simulink model "UpgradedConveyorBeltMechanism"  (R2023a)
settings: Solver=VariableStepAuto  StartTime=0.0  StopTime=30  RelTol=1e-3
values from neighbouring files (symbols this model uses):
  b = 40.6518    [UpgradedConveyorBeltParameters.m]
  B1 = 0.0042    [UpgradedConveyorBeltParameters.m]
  B2 = 0.0084    [UpgradedConveyorBeltParameters.m]
  J1 = 7e-5    (= 7e-05)    [UpgradedConveyorBeltParameters.m]
  J2 = 8e-5    (= 8e-05)    [UpgradedConveyorBeltParameters.m]
  k1 = 2.6552e5    (= 265520)    [UpgradedConveyorBeltParameters.m]
  k2 = 2.6552e5    (= 265520)    [UpgradedConveyorBeltParameters.m]
  k3 = 11.777e4    (= 117770)    [UpgradedConveyorBeltParameters.m]
  Kb = 23e-3    (= 0.023)    [UpgradedConveyorBeltParameters.m]
  Kt = 23e-3    (= 0.023)    [UpgradedConveyorBeltParameters.m]
  L = 0.1    [UpgradedConveyorBeltParameters.m]
  m = 2    [UpgradedConveyorBeltParameters.m]
  R = 0.71    [UpgradedConveyorBeltParameters.m]
  r = 0.0194    [UpgradedConveyorBeltParameters.m]
undefined symbols (not defined in the file or in its folder): J, Kd, Ke
libraries: fl_lib x20, slpidlib x10, fl_ps_legacy_lib x8, nesl_utility x6, SignalEditorBlockLib x5, ee_lib x2, simulink x1
(part 1 of 2)
settings Model: PacingRate=10  Creator=M3tal  LastModifiedBy=M3tal
settings OptimizationCC: DefaultParameterBehavior=Inlined  EnhancedBackFolding=on  PassReuseOutputArgsThreshold=0  OptimizeBlockOrder=speed  DifferentSizesBufferReuse=on
settings DebuggingCC: ParameterTunabilityLossMsg=error
settings HardwareCC: TargetBitPerPointer=64  TargetBitPerSizeT=64  TargetBitPerPtrDiffT=64  TargetLongLongMode=on  TargetIntDivRoundTo=Zero  TargetEndianess=LittleEndian  TargetWordSize=64  TargetHWDeviceType=MATLAB Host  ProdEqTarget=off
settings SFSimCC: MATLABDynamicMemAlloc=off
settings RTWCC: GenCodeOnly=on
settings CodeAppCC: ForceParamTrailComments=on  OperatorAnnotations=on

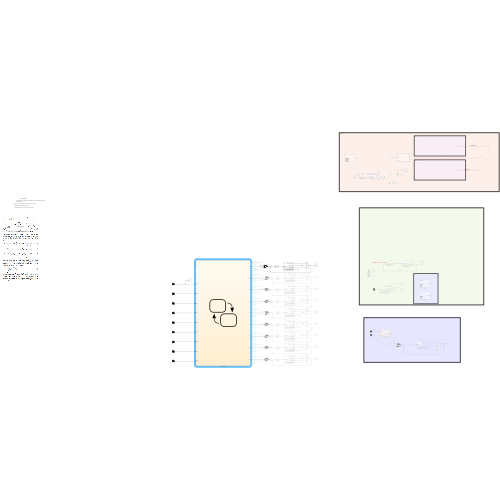
[thumbnail: Simulink's stored preview of the top-level diagram]
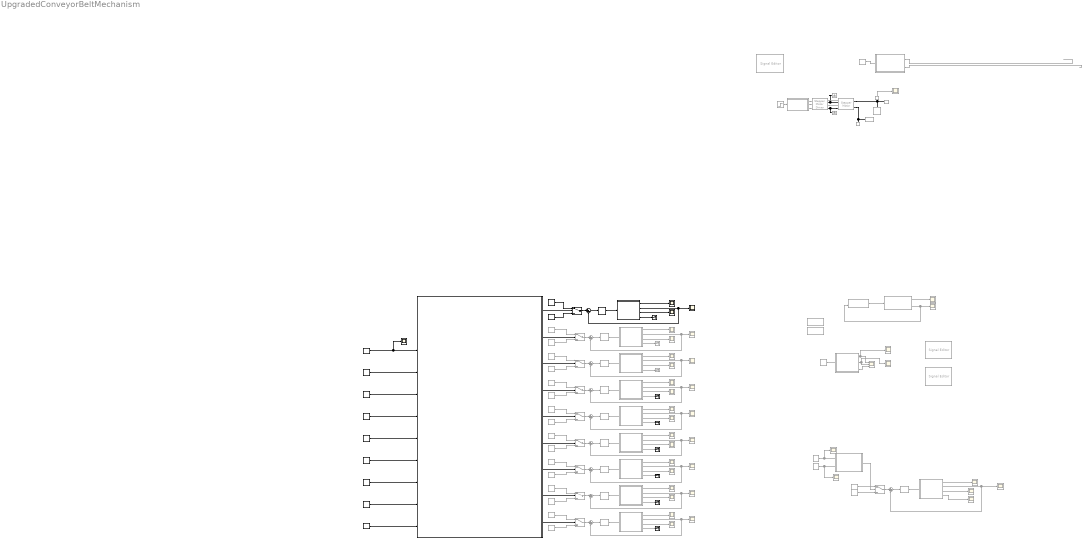
== system UpgradedConveyorBeltMechanism ==
  note: Steppers
  note: X-axis
  note: -replace signals with inports and outports
  note: -record the speed of the dc motor over a period of time
  note: -caluclating the number of steps for each motor for each meal
  note: Y-axis
  note: we using the same mechansim for the steppers that convert the rotational motion to translational motion
  note: m=r*angle in radians
  Belt Mechanism10 : Subsystem  Commented=on
  Constant{,5,7,9,11,13,15,17,19} (9 alike) : Constant  Commented=on  Value=0.2
  Constant{1,6,8,10,12,14,16,18,20} (9 alike) : Constant  Commented=on  Value=0
  Constant2 : Constant  Commented=on
  Constant3 : Constant  Value=0.2
  Constant4 : Constant  Value=0
  Controller : Subsystem  Commented=on  Variant=on  VariantControlMode=label  LabelModeActiveChoice=Position
      settings: AttributesFormatString=%<BlockChoice>
  DC Motor10 : Subsystem  Commented=on
  Demand : Step  Commented=on  Before=10  After=0  SampleTime=0
  ERef A+ : fl_lib/Electrical/Electrical Elements/Electrical Reference  Commented=on
  ERef B- : fl_lib/Electrical/Electrical Elements/Electrical Reference  Commented=on
  Inertia1 : fl_lib/Mechanical/Rotational Elements/Inertia  Commented=on  inertia=0.1 kg*m^2  num_ports=foundation.enum.numPorts2.one  w_specify=off  w_priority=High  w=0 rad/s  w_nominal_specify=off  w_nominal_unit=rad/s  w_nominal_value=1  t_specify=off  t_priority=None  t=0 N*m  t_nominal_specify=off  t_nominal_unit=N*m  t_nominal_value=1
  MATLAB Function : MATLAB Function  Commented=on  TreatAsAtomicUnit=on
  MRRef Motor : fl_lib/Mechanical/Rotational Elements/Mechanical Rotational Reference  Commented=on
  PID Controller{,2..9} (9 alike) : slpidlib/PID Controller  Commented=on  Controller=PID  Form=Parallel  TimeDomain=Continuous-time  UseExternalTs=off  SampleTime=-1  IntegratorMethod=Forward Euler  FilterMethod=Forward Euler  ControllerParametersSource=internal  P=29.8496571480823  I=152.933850283855  UseKiTs=off  D=-0.451147774638306  N=4.48716691500189  UseFilter=on  TunerSelectOption=Transfer Function Based (PID Tuner App)  InitialConditionSource=internal  InitialConditionForIntegrator=0  InitialConditionForFilter=0  DifferentiatorICPrevScaledInput=0  ExternalReset=none  TrackingMode=off  Kt=1  LimitOutput=off  SatLimitsSource=internal  UpperSaturationLimit=inf  LowerSaturationLimit=-inf  LinearizeAsGain=on  AntiWindupMode=none  Kb=1  LimitIntegrator=off  UpperIntegratorSaturationLimit=inf  LowerIntegratorSaturationLimit=-inf  POutMin=[]  POutMax=[]  IOutMin=[]  IOutMax=[]  DOutMin=[]  DOutMax=[]  NOutMin=[]  NOutMax=[]  SumOutMin=[]  SumOutMax=[]  SaturationOutMin=[]  SaturationOutMax=[]  PParamMin=[]  PParamMax=[]  IParamMin=[]  IParamMax=[]  DParamMin=[]  DParamMax=[]  NParamMin=[]  NParamMax=[]  KbParamMin=[]  KbParamMax=[]  KtParamMin=[]  KtParamMax=[]  KbOutMin=[]  KbOutMax=[]  KtOutMin=[]  KtOutMax=[]  IntegratorOutMin=[]  IntegratorOutMax=[]  FilterOutMin=[]  FilterOutMax=[]  SumI1OutMin=[]  SumI1OutMax=[]  SumI2OutMin=[]  SumI2OutMax=[]  SumI3OutMin=[]  SumI3OutMax=[]  SumI4OutMin=[]  SumI4OutMax=[]  SumDOutMin=[]  SumDOutMax=[]  DifferentiatorOutMin=[]  DifferentiatorOutMax=[]  FilterDiffOutCoefMin=[]  FilterDiffOutCoefMax=[]  ReciprocalOutMin=[]  ReciprocalOutMax=[]  SumDenOutMin=[]  SumDenOutMax=[]  SumNumOutMin=[]  SumNumOutMax=[]  DivideOutMin=[]  DivideOutMax=[]  UdiffTsProdOutMin=[]  UdiffTsProdOutMax=[]  NTsProdOutMin=[]  NTsProdOutMax=[]  UintegralTsProdOutMin=[]  UintegralTsProdOutMax=[]  UngainTsProdOutMin=[]  UngainTsProdOutMax=[]  ClampingZeroOutDataTypeStr=Inherit: Inherit via back propagation  ClampingZeroOutMin=[]  ClampingZeroOutMax=[]  FilterDenConstantOutDataTypeStr=Inherit: Inherit via back propagation  FilterDenConstantOutMin=[]  FilterDenConstantOutMax=[]  PCopyOutDataTypeStr=Inherit: Inherit via back propagation  PCopyOutMin=[]  PCopyOutMax=[]  NCopyOutDataTypeStr=Inherit: Inherit via back propagation  NCopyOutMin=[]  NCopyOutMax=[]  IntegratorContinuousStateAttributes=''  IntegratorStateMustResolveToSignalObject=off  IntegratorRTWStateStorageClass=Auto  FilterContinuousStateAttributes=''  FilterStateMustResolveToSignalObject=off  FilterRTWStateStorageClass=Auto  ParallelPVariant=InternalParameters  IdealPVariant=Disabled  IVariant=InternalParameters  DVariant=InternalParameters  IntegratorVariant=Continuous  SatVariant=Disabled  AWVariant=Passthrough  PCopyVariant=Disabled  TRVariant=Disabled  FdbkBlocksVariant=Forward  IdealPFdbkVariant=Disabled  SatFdbkVariant=Disabled  DerivativeFilterVariant=ContFilter  NVariant=InternalParameters  NCopyVariant=Disabled  FilterICVariant=InternalICsFilter  IntegratorICVariant=InternalICs  ExternalResetVariant=Disabled  TRSumVariant=Passthrough  SumFdbkVariant=Disabled  SumVariant=Sum_PID  TsampFilterVariant=InternalTs  TsampNgainVariant=Passthrough  TsampIntegralVariant=Disabled_SignalSpec  ExternalSaturationOutDataTypeStr=Inherit: Same as second input
  PID Controller1 : slpidlib/PID Controller  Controller=PID  Form=Parallel  TimeDomain=Continuous-time  UseExternalTs=off  SampleTime=-1  IntegratorMethod=Forward Euler  FilterMethod=Forward Euler  ControllerParametersSource=internal  P=29.8496571480823  I=152.933850283855  UseKiTs=off  D=-0.451147774638306  N=4.48716691500189  UseFilter=on  TunerSelectOption=Transfer Function Based (PID Tuner App)  InitialConditionSource=internal  InitialConditionForIntegrator=0  InitialConditionForFilter=0  DifferentiatorICPrevScaledInput=0  ExternalReset=none  TrackingMode=off  Kt=1  LimitOutput=off  SatLimitsSource=internal  UpperSaturationLimit=inf  LowerSaturationLimit=-inf  LinearizeAsGain=on  AntiWindupMode=none  Kb=1  LimitIntegrator=off  UpperIntegratorSaturationLimit=inf  LowerIntegratorSaturationLimit=-inf  POutMin=[]  POutMax=[]  IOutMin=[]  IOutMax=[]  DOutMin=[]  DOutMax=[]  NOutMin=[]  NOutMax=[]  SumOutMin=[]  SumOutMax=[]  SaturationOutMin=[]  SaturationOutMax=[]  PParamMin=[]  PParamMax=[]  IParamMin=[]  IParamMax=[]  DParamMin=[]  DParamMax=[]  NParamMin=[]  NParamMax=[]  KbParamMin=[]  KbParamMax=[]  KtParamMin=[]  KtParamMax=[]  KbOutMin=[]  KbOutMax=[]  KtOutMin=[]  KtOutMax=[]  IntegratorOutMin=[]  IntegratorOutMax=[]  FilterOutMin=[]  FilterOutMax=[]  SumI1OutMin=[]  SumI1OutMax=[]  SumI2OutMin=[]  SumI2OutMax=[]  SumI3OutMin=[]  SumI3OutMax=[]  SumI4OutMin=[]  SumI4OutMax=[]  SumDOutMin=[]  SumDOutMax=[]  DifferentiatorOutMin=[]  DifferentiatorOutMax=[]  FilterDiffOutCoefMin=[]  FilterDiffOutCoefMax=[]  ReciprocalOutMin=[]  ReciprocalOutMax=[]  SumDenOutMin=[]  SumDenOutMax=[]  SumNumOutMin=[]  SumNumOutMax=[]  DivideOutMin=[]  DivideOutMax=[]  UdiffTsProdOutMin=[]  UdiffTsProdOutMax=[]  NTsProdOutMin=[]  NTsProdOutMax=[]  UintegralTsProdOutMin=[]  UintegralTsProdOutMax=[]  UngainTsProdOutMin=[]  UngainTsProdOutMax=[]  ClampingZeroOutDataTypeStr=Inherit: Inherit via back propagation  ClampingZeroOutMin=[]  ClampingZeroOutMax=[]  FilterDenConstantOutDataTypeStr=Inherit: Inherit via back propagation  FilterDenConstantOutMin=[]  FilterDenConstantOutMax=[]  PCopyOutDataTypeStr=Inherit: Inherit via back propagation  PCopyOutMin=[]  PCopyOutMax=[]  NCopyOutDataTypeStr=Inherit: Inherit via back propagation  NCopyOutMin=[]  NCopyOutMax=[]  IntegratorContinuousStateAttributes=''  IntegratorStateMustResolveToSignalObject=off  IntegratorRTWStateStorageClass=Auto  FilterContinuousStateAttributes=''  FilterStateMustResolveToSignalObject=off  FilterRTWStateStorageClass=Auto  ParallelPVariant=InternalParameters  IdealPVariant=Disabled  IVariant=InternalParameters  DVariant=InternalParameters  IntegratorVariant=Continuous  SatVariant=Disabled  AWVariant=Passthrough  PCopyVariant=Disabled  TRVariant=Disabled  FdbkBlocksVariant=Forward  IdealPFdbkVariant=Disabled  SatFdbkVariant=Disabled  DerivativeFilterVariant=ContFilter  NVariant=InternalParameters  NCopyVariant=Disabled  FilterICVariant=InternalICsFilter  IntegratorICVariant=InternalICs  ExternalResetVariant=Disabled  TRSumVariant=Passthrough  SumFdbkVariant=Disabled  SumVariant=Sum_PID  TsampFilterVariant=InternalTs  TsampNgainVariant=Passthrough  TsampIntegralVariant=Disabled_SignalSpec  ExternalSaturationOutDataTypeStr=Inherit: Same as second input
  Pulse Generator : DiscretePulseGenerator  Commented=on  PulseType=Time based  Period=40  PhaseDelay=20
  Pulse Generator1 : DiscretePulseGenerator  Commented=on  PulseType=Time based  Period=50  PhaseDelay=5
  Pulse Generator{3..10} (8 alike) : DiscretePulseGenerator  PulseType=Time based  Amplitude=0  Period=50  PhaseDelay=5
  Pulse Generator11 : DiscretePulseGenerator  Commented=on  PulseType=Time based  Amplitude=12  Period=11  PulseWidth=50  PhaseDelay=2
  Pulse Generator2 : DiscretePulseGenerator  PulseType=Time based  Period=50  PulseWidth=50  PhaseDelay=25
  Scope{,1..3,8..22,24..38} (34 alike) : Scope  Commented=on
  Scope23 : Scope  Commented=on  NumInputPorts=3
  Scope{4..7} (4 alike) : Scope
  Sensing Angle : Subsystem  Commented=on
      mask Display: disp('a')
  Sensor : SignalEditorBlockLib/Signal Editor  Commented=on  FileName=Crane_Sensor.mat  ActiveScenario=Scenario  ActiveSignal=Crane signal  IsBus=off  OutputBusObjectStr=Bus: BusObject  SampleTime=0  Interpolate=off  ZeroCross=off  OutputAfterFinalValue=Setting to zero  Unit=inherit  PreserveSignalName=on  ApplySigPropsToAllScenarios=on
  Sensor1 : SignalEditorBlockLib/Signal Editor  Commented=on  FileName=Belt_Sensor.mat  ActiveScenario=Scenario  ActiveSignal=Belt Signal  IsBus=off  OutputBusObjectStr=Bus: BusObject  SampleTime=0  Interpolate=off  ZeroCross=off  OutputAfterFinalValue=Setting to zero  Unit=inherit  PreserveSignalName=on  ApplySigPropsToAllScenarios=on
  Sensors : Stateflow chart  Commented=on  TreatAsAtomicUnit=on
  Sensors Logic : Stateflow chart  TreatAsAtomicUnit=on
      settings: PortSchema="{\"entries\":[{\"content\":{\"sides\":[{\"content\":{\"connectorIds\":[\"In10\",\"In11\",\"In1\",\"In2\",\"In3\",\"In4\",\"In5\",\"In6\",\"In7\",\"In8\",\"In9\"]},\"type\":\"ConnectorPlacement.EquallySpacedRectSide\",\"uuid\":\"dd9ce701-3689-4654-9b21-5529dab0541a\"},{\"content\":{\"connectorIds\":[\"Out1\",\"Out2\",\"Out3\",\"Out4\",\"Out5\",\"Out6\",\"Out7\",\"Out8\",\"Out9\"],\"side\":\"RIGHT\"},\"type\":\"ConnectorPlacement.EquallySpacedRectSide\",\"uuid\":\"ff8f0f67-846c-4703-aeda-d87216d47c92\"},{\"content\":{\"side\":\"TOP\"},\"type\":\"ConnectorPlacement.EquallySpacedRectSide\",\"uuid\":\"ae968bb7-da0f-44fd-802b-06f57922bbce\"}]},\"type\":\"ConnectorPlacement.EquallySpacedConnector\",\"uuid\":\"820653e5-881f-4b8b-9810-894dc5dde637\"}],\"packageUris\":[\"http://schema.mathworks.com/mf0/Connector/R2020b\"],\"version\":\"1.0\"}"
  Shaft Angle : Scope  Commented=on
  Shaft Free End : fl_lib/Mechanical/Rotational Elements/Rotational Free End  Commented=on  w_specify=off  w_priority=None  w=0 rad/s  w_nominal_specify=off  w_nominal_unit=rad/s  w_nominal_value=1
  Signal Editor : SignalEditorBlockLib/Signal Editor  Commented=on  FileName=X_Position.mat  ActiveScenario=Scenario  ActiveSignal=X  IsBus=off  OutputBusObjectStr=Bus: BusObject  SampleTime=0  Interpolate=off  ZeroCross=off  OutputAfterFinalValue=Setting to zero  Unit=inherit  PreserveSignalName=on  ApplySigPropsToAllScenarios=on
  Signal Editor1 : SignalEditorBlockLib/Signal Editor  Commented=on  FileName=Y_Position.mat  ActiveScenario=Scenario  ActiveSignal=Y  IsBus=off  OutputBusObjectStr=Bus: BusObject  SampleTime=0  Interpolate=off  ZeroCross=off  OutputAfterFinalValue=Setting to zero  Unit=inherit  PreserveSignalName=on  ApplySigPropsToAllScenarios=on
  Signal Editor2 : SignalEditorBlockLib/Signal Editor  Commented=on  FileName=untitled.mat  ActiveScenario=Scenario  ActiveSignal=Signal 1  IsBus=off  OutputBusObjectStr=Bus: BusObject  SampleTime=0  Interpolate=off  ZeroCross=off  OutputAfterFinalValue=Setting to zero  Unit=inherit  PreserveSignalName=on  ApplySigPropsToAllScenarios=on
  Solver Configuration : nesl_utility/Solver Configuration  Commented=on  PhysicalDomain=network_engine_domain  SubClassName=solver  LeftPortType=input  RightPortType=generic  Tones=[]  Harmonics=[]  SimulateNoise=off  Profile=off  UseLocalSampling=off  EnableSwitchedLinearOptims=on  FrequencyDomain=off  UseCCode=off  RelTol=0.001  AbsTol=1e-06  MinStep=1e-09  ToWorkspace=off  RevertToSquareIcSolve=off  NumHomotopyIterations=100  PhasorMode=off  PhasorModeNumHarmonics=1  ConsistencySolver=NEWTON_FTOL  IndexReductionMethod=DerivativeReplacement  DoDC=off  ResidualTolerance=1e-9  ConsistencyTolSource=GLOBAL  ConsistencyAbsTol=0.001  ConsistencyRelTol=0.001  ConsistencyTolFactor=0.001  UseLocalSolver=off  LocalSolverChoice=NE_BACKWARD_EULER_ADVANCER  ResolveIndetEquations=on  FunctionEvalNumThread=1  LocalSolverSampleTime=.001  DoFixedCost=off  MaxNonlinIter=3  MaxModeIter=2  ComputeImpulses=off  ImpulseIterations=2  LinearAlgebra=auto  LinearAlgebraNumThread=0  EquationFormulation=NE_TIME_EF  DelaysMemoryBudget=1024  AutomaticFiltering=on  FilteringTimeConstant=0.001  PartitionStorageMethod=AS_NEEDED  PartitionMemoryBudget=1024  PartitionMethod=FAST
  Stepper Motor : ee_lib/Electromechanical/Reluctance & Stepper/Stepper Motor  Commented=on  step_or_av=ee.enum.electromech.simulationMode.stepping  Ra=1.3 Ohm  La=2.9 mH  Km=0.315 N*m/A  Td=25 mN*m  Rm=Inf Ohm  w_vec=[ 0 1000 3e+3 ] rpm  T_vec=[ 2 2 1 ] N*m  assert_if_slipping=0  J_total=1e-4 kg*m^2  max_step_rate=10 Hz  Step=1.8 deg  J=82 g*cm^2  B=1e-2 N*m/(rad/s)  speed0=0 rpm  theta0=0 deg  alpha=[.00393, .00393] 1/K  Tmeas=25 degC  Tmeas2=125 degC  T_vec2=[1.7, 1.7, .85] N*m  half_stepping=ee.enum.electromech.steppingModeAveraged.fullStep  thermal_masses=[100, 100] J/K  initial_temperatures=[25, 25] degC  rotor_thermal_mass=50 J/K  rotor_initial_temperature=25 degC  Rm_percent_rotor=90
      settings: InternalSimscapePortConfiguration="{\"Bottom\":[],\"Left\":[{\"id\":\"pA\",\"label\":\"A+\",\"type\":\"foundation.electrical.electrical\"},{\"id\":\"nA\",\"label\":\"A-\",\"type\":\"foundation.electrical.electrical\"},{\"id\":\"pB\",\"label\":\"B+\",\"type\":\"foundation.electrical.electrical\"},{\"id\":\"nB\",\"label\":\"B-\",\"type\":\"foundation.electrical.electrical\"}],\"Right\":[{\"id\":\"R\",\"label\":\"R\",\"type\":\"foundation.mechanical.rotational.rotational\"},{\"id\":\"C\",\"label\":\"C\",\"type\":\"foundation.mechanical.rotational.rotational\"}],\"Top\":[]}"
  Stepper Motor Driver : ee_lib/Electromechanical/Reluctance & Stepper/Stepper Motor Driver  Commented=on  step_or_av=1  step_rate_per_volt=10 Hz/V  Venable=2.5 V  Vreverse=2.5 V  supply_ports=ee.enum.supply_ports.hidesupply  Vm=5 V  Vsupply=10 V  half_stepping=0  stepping_mode=ee.enum.electromech.steppingMode.fullStep  numMicroSteps=4  Im=1.2 A
      settings: InternalSimscapePortConfiguration="{\"Bottom\":[],\"Left\":[{\"id\":\"ENA\",\"label\":\"ENA\",\"type\":\"foundation.electrical.electrical\"},{\"id\":\"REF\",\"label\":\"REF\",\"type\":\"foundation.electrical.electrical\"},{\"id\":\"REV\",\"label\":\"REV\",\"type\":\"foundation.electrical.electrical\"}],\"Right\":[{\"id\":\"pA\",\"label\":\"A+\",\"type\":\"foundation.electrical.electrical\"},{\"id\":\"nA\",\"label\":\"A-\",\"type\":\"foundation.electrical.electrical\"},{\"id\":\"pB\",\"label\":\"B+\",\"type\":\"foundation.electrical.electrical\"},{\"id\":\"nB\",\"label\":\"B-\",\"type\":\"foundation.electrical.electrical\"}],\"Top\":[]}"
  Subsystem : Subsystem  Commented=on
  Subsystem1 : Subsystem  Commented=on
  Subsystem10 : Subsystem  Commented=on
  Subsystem2 : Subsystem
  Subsystem3 : Subsystem  Commented=on
  Subsystem4 : Subsystem  Commented=on
  Subsystem5 : Subsystem  Commented=on
  Subsystem6 : Subsystem  Commented=on
  Subsystem7 : Subsystem  Commented=on
  Subsystem8 : Subsystem  Commented=on
  Subsystem9 : Subsystem  Commented=on
  Sum{,2..9} (9 alike) : Sum  Commented=on  Inputs=|+-
  Sum1 : Sum  Inputs=|+-
  Switch{,2..9} (9 alike) : Switch  Commented=on  Criteria=u2 ~= 0  Threshold=1  SaturateOnIntegerOverflow=off  InputSameDT=off
  Switch1 : Switch  Criteria=u2 ~= 0  Threshold=1  SaturateOnIntegerOverflow=off  InputSameDT=off
  Terminator{,3..8} (7 alike) : Terminator
  Terminator1 : Terminator  Commented=on
  Terminator2 : Terminator  Commented=on
  wires:
  Pulse Generator1/1 -> Scope/1, Sensors/1(Crane)
  Subsystem1/2(load velocity) -> Sum/2, Scope2/1  "Velocity"
  Pulse Generator/1 -> Scope3/1, Sensors/2(Belt)
  Subsystem/1(drive pulley velocity) -> Scope25/1, Scope23/1
  Subsystem/2(load velocity) -> Scope23/2, Scope24/1
  Subsystem/3(driven pulley velocity) -> Scope23/3
  Pulse Generator11/1 -> Subsystem/1(Voltage)
  Sum/1 -> PID Controller/1
  Sensors/1(Voltage) -> Switch/2
  Constant1/1 -> Switch/3
  PID Controller/1 -> Subsystem1/1(Voltage)
  Switch/1 -> Sum/1
  Constant/1 -> Switch/1
  Subsystem1/1(drive pulley velocity) -> Scope26/1
  Subsystem1/4(driven pulley Velocity) -> Scope27/1
  Subsystem1/3(load position) -> Scope1/1
  Pulse Generator5/1 -> Sensors Logic/4(Belt4)
  Pulse Generator9/1 -> Sensors Logic/8(Belt8)
  Pulse Generator7/1 -> Sensors Logic/6(Belt6)
  Pulse Generator2/1 -> Scope4/1, Sensors Logic/1(Belt1)
  Pulse Generator8/1 -> Sensors Logic/7(Belt7)
  Pulse Generator3/1 -> Sensors Logic/2(Belt2)
  Pulse Generator6/1 -> Sensors Logic/5(Belt5)
  Pulse Generator10/1 -> Sensors Logic/9(Belt9)
  Pulse Generator4/1 -> Sensors Logic/3(Belt3)
  Constant2/1 -> MATLAB Function/1(meal)
  ? -> DC Motor10/1(Voltage)
  Belt Mechanism10/2(Velocity) -> Scope29/1, DC Motor10/2(Velocity)  "Velocity"
  Belt Mechanism10/1(Position) -> Scope28/1
  DC Motor10/1(Tourque) -> Belt Mechanism10/1(Tourque)  "Tourque"
  Subsystem2/1(drive pulley velocity) -> Scope7/1
  Sum1/1 -> PID Controller1/1
  Switch1/1 -> Sum1/1
  Constant3/1 -> Switch1/1
  Constant4/1 -> Switch1/3
  PID Controller1/1 -> Subsystem2/1(Voltage)
  Subsystem2/2(load velocity) -> Sum1/2, Scope6/1  "Velocity"
  Subsystem2/3(load position) -> Scope5/1
  Subsystem2/4(driven pulley Velocity) -> Terminator/1
  Sensors Logic/1(V1) -> Switch1/2
  Subsystem3/3(load position) -> Scope8/1
  Sensors Logic/2(V2) -> Switch2/2
  Sum2/1 -> PID Controller2/1
  Constant6/1 -> Switch2/3
  Subsystem3/1(drive pulley velocity) -> Scope10/1
  Subsystem3/2(load velocity) -> Sum2/2, Scope9/1  "Velocity"
  PID Controller2/1 -> Subsystem3/1(Voltage)
  Constant5/1 -> Switch2/1
  Switch2/1 -> Sum2/1
  Subsystem3/4(driven pulley Velocity) -> Terminator1/1
  Subsystem4/4(driven pulley Velocity) -> Terminator2/1
  Sum3/1 -> PID Controller3/1
  Constant8/1 -> Switch3/3
  Subsystem4/2(load velocity) -> Sum3/2, Scope13/1  "Velocity"
  Switch3/1 -> Sum3/1
  Constant7/1 -> Switch3/1
  PID Controller3/1 -> Subsystem4/1(Voltage)
  Subsystem4/3(load position) -> Scope12/1
  Subsystem4/1(drive pulley velocity) -> Scope11/1
  Sensors Logic/3(V3) -> Switch3/2
  Subsystem5/4(driven pulley Velocity) -> Terminator3/1
  Sum4/1 -> PID Controller4/1
  Constant10/1 -> Switch4/3
  Subsystem5/2(load velocity) -> Sum4/2, Scope16/1  "Velocity"
  Switch4/1 -> Sum4/1
  Constant9/1 -> Switch4/1
  PID Controller4/1 -> Subsystem5/1(Voltage)
  Subsystem5/3(load position) -> Scope15/1
  Subsystem5/1(drive pulley velocity) -> Scope14/1
  Sensors Logic/4(V4) -> Switch4/2
  Subsystem6/4(driven pulley Velocity) -> Terminator4/1
  Sum5/1 -> PID Controller5/1
  Constant12/1 -> Switch5/3
  Subsystem6/2(load velocity) -> Sum5/2, Scope19/1  "Velocity"
  Switch5/1 -> Sum5/1
  Constant11/1 -> Switch5/1
  PID Controller5/1 -> Subsystem6/1(Voltage)
  Subsystem6/3(load position) -> Scope18/1
  Subsystem6/1(drive pulley velocity) -> Scope17/1
  Sensors Logic/5(V5) -> Switch5/2
  Sensors Logic/6(V6) -> Switch6/2
  Subsystem7/1(drive pulley velocity) -> Scope20/1
  Subsystem7/2(load velocity) -> Sum6/2, Scope22/1  "Velocity"
  Subsystem7/3(load position) -> Scope21/1
  Subsystem7/4(driven pulley Velocity) -> Terminator5/1
  Constant13/1 -> Switch6/1
  Switch6/1 -> Sum6/1
  Constant14/1 -> Switch6/3
  Sum6/1 -> PID Controller6/1
  PID Controller6/1 -> Subsystem7/1(Voltage)
  Sensors Logic/7(V7) -> Switch7/2
  Subsystem8/1(drive pulley velocity) -> Scope30/1
  Sum7/1 -> PID Controller7/1
  Constant16/1 -> Switch7/3
  Subsystem8/2(load velocity) -> Sum7/2, Scope32/1  "Velocity"
  Subsystem8/4(driven pulley Velocity) -> Terminator6/1
  Constant15/1 -> Switch7/1
  Subsystem8/3(load position) -> Scope31/1
  Switch7/1 -> Sum7/1
  PID Controller7/1 -> Subsystem8/1(Voltage)
  PID Controller8/1 -> Subsystem9/1(Voltage)
  Switch8/1 -> Sum8/1
  Constant17/1 -> Switch8/1
  Subsystem9/3(load position) -> Scope34/1
  Subsystem9/1(drive pulley velocity) -> Scope33/1
  Subsystem9/4(driven pulley Velocity) -> Terminator7/1
  Sum8/1 -> PID Controller8/1
  Subsystem9/2(load velocity) -> Sum8/2, Scope35/1  "Velocity"
  Sensors Logic/8(V8) -> Switch8/2
  Constant18/1 -> Switch8/3
  Subsystem10/2(load velocity) -> Sum9/2, Scope38/1  "Velocity"
  Constant20/1 -> Switch9/3
  Subsystem10/1(drive pulley velocity) -> Scope36/1
  Subsystem10/3(load position) -> Scope37/1
  Subsystem10/4(driven pulley Velocity) -> Terminator8/1
  Sum9/1 -> PID Controller9/1
  PID Controller9/1 -> Subsystem10/1(Voltage)
  Sensors Logic/9(V9) -> Switch9/2
  Switch9/1 -> Sum9/1
  Constant19/1 -> Switch9/1
  ? -> ?  "XTheta (degrees)"
  ? -> ?  "YTheta (degrees)"
  Demand/1 -> Controller/1(Ref)
  Sensing Angle/1(theta) -> Shaft Angle/1
  MATLAB Function/1(x) -> ?
  MATLAB Function/2(y) -> ?
  connections:
  MRRef Motor/LConn1 -- Stepper Motor/RConn2 -- Solver Configuration/RConn1
  Stepper Motor/LConn4 -- Stepper Motor Driver/RConn4 -- ERef B-/LConn1
  Stepper Motor Driver/RConn2 -- Stepper Motor/LConn2 -- ERef A+/LConn1
  Sensing Angle/LConn1 -- Stepper Motor/RConn1 -- Inertia1/LConn1 -- Shaft Free End/LConn1
  Stepper Motor Driver/RConn1 -- Stepper Motor/LConn1
  Controller/RConn2 -- Stepper Motor Driver/LConn2
  Controller/RConn3 -- Stepper Motor Driver/LConn3
  Controller/RConn1 -- Stepper Motor Driver/LConn1
  Stepper Motor Driver/RConn3 -- Stepper Motor/LConn3

== system UpgradedConveyorBeltMechanism/Belt Mechanism10 ==
  note: Note: The term $K \frac{d\theta}{dt}$ ​ represents a damping torque that is proportional to the angular velocity
  note: $\frac{d^2\theta}{dt^2} = \frac{1}{J} \left(T - K \frac{d\theta}{dt}\right)$
      | belt mechanism equaition based on newton seconed law for rotational motion
  Tourque : Inport
  Gain1 : Gain  Gain=1/J
  Integrator2 : Integrator
  Integrator3 : Integrator
  Subtract : Sum  Inputs=+-
  damping coefficient : Gain  Gain=Kd
  Position : Outport
  Velocity : Outport  Port=2
  wires:
  Integrator2/1 -> damping coefficient/1, Velocity/1, Integrator3/1  "Velocity"
  Tourque/1 -> Subtract/1
  Subtract/1 -> Gain1/1
  Integrator3/1 -> Position/1  "Position"
  damping coefficient/1 -> Subtract/2
  Gain1/1 -> Integrator2/1  "theta_dot_dot"

== system UpgradedConveyorBeltMechanism/Controller ==
  Ref : Inport
  Position : Subsystem  VariantControl=Position
  Speed : Subsystem  VariantControl=Speed
  PWM : PMIOPort  Side=Right
  0v : PMIOPort  Port=2  Side=Right
  REV : PMIOPort  Port=3  Side=Right

== system UpgradedConveyorBeltMechanism/DC Motor10 ==
  note: Armature Controlled DC Motor
      |
      | $E_a = R_a \cdot I_a + L_a \cdot \frac{di_a}{dt} + K_b \cdot \frac{d\theta}{dt}$
      | $T_{m} = K_{t} \cdot I_{a}$
  Voltage : Inport
  Velocity : Inport  Port=2
  Constant1 : Constant  Value=R
  Gain1 : Gain  Gain=Kb
  Gain2 : Gain  Gain=1/L
  Gain3 : Gain  Gain=Kt
  Integrator : Integrator
  Product : Product
  Subtract : Sum  Inputs=+--
  Tourque : Outport
  wires:
  Voltage/1 -> Subtract/1
  Integrator/1 -> Product/1, Gain3/1  "i"
  Gain3/1 -> Tourque/1
  Gain1/1 -> Subtract/2
  Velocity/1 -> Gain1/1
  Constant1/1 -> Product/2
  Product/1 -> Subtract/3
  Gain2/1 -> Integrator/1  "i_dot"
  Subtract/1 -> Gain2/1

== system UpgradedConveyorBeltMechanism/Sensing Angle ==
  MRRef : fl_lib/Mechanical/Rotational Elements/Mechanical Rotational Reference
  Motion Sensor : fl_lib/Mechanical/Mechanical Sensors/Ideal Rotational Motion Sensor  reference=foundation.enum.MeasurementReference.difference  acceleration_port=false  velocity_port=true  position_port=true  wrap_angle=simscape.enum.onoff.off  offset=0 rad
  deg : nesl_utility/PS-Simulink Converter  PhysicalDomain=network_engine_domain  SubClassName=ps_output  LeftPortType=input  RightPortType=output  PseudoPeriodic=off  Frequencies=[]  VectorFormat=1-D array  Unit=deg  AffineConversion=off
  R : PMIOPort  Side=Left
  theta : Outport  VectorParamsAs1DForOutWhenUnconnected=off
  wires:
  deg/1 -> theta/1
  connections:
  R/RConn1 -- Motion Sensor/LConn1
  Motion Sensor/RConn3 -- deg/LConn1
  MRRef/LConn1 -- Motion Sensor/RConn1

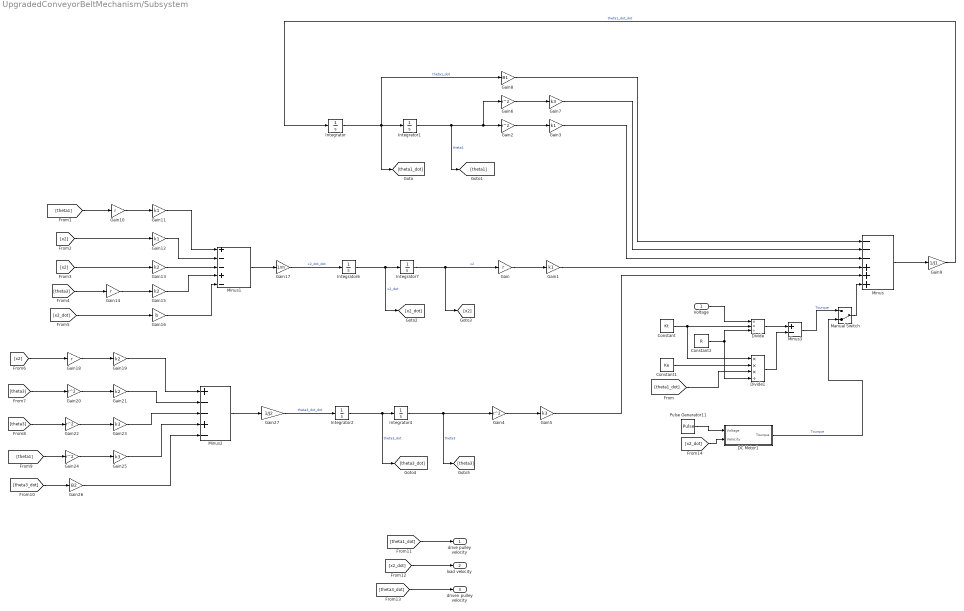
== system UpgradedConveyorBeltMechanism/Subsystem ==
  Voltage : Inport
  Constant : Constant  Value=Kt
  Constant1 : Constant  Value=Ke
  Constant2 : Constant  Value=R
  DC Motor1 : Subsystem
  Divide : Product  Inputs=**/
  Divide1 : Product  Inputs=***/
  Gain{,10,14,18} (4 alike) : Gain  Gain=r
  Gain{1,3,11..12} (4 alike) : Gain  Gain=k1
  Gain{13,15,19,21} (4 alike) : Gain  Gain=k2
  Gain16 : Gain  Gain=b
  Gain17 : Gain  Gain=1/m
  Gain{2,4,6,20,22,24} (6 alike) : Gain  Gain=r^2
  Gain{5,7,23,25} (4 alike) : Gain  Gain=k3
  Gain26 : Gain  Gain=B2
  Gain27 : Gain  Gain=1/J2
  Gain8 : Gain  Gain=B1
  Gain9 : Gain  Gain=1/J1
  Integrator{,1..2,4,6..7} (6 alike) : Integrator
  Manual Switch : ManualSwitch  CurrentSetting=0
  Minus : Sum  Inputs=---+++
  Minus1 : Sum  Inputs=+--+-
  Minus2 : Sum  Inputs=+--+-
  Minus3 : Sum  Inputs=+-
  Pulse Generator11 : DiscretePulseGenerator  PulseType=Time based  Amplitude=12  Period=11  PulseWidth=50  PhaseDelay=2
  drive pulley velocity : Outport
  load velocity : Outport  Port=2
  driven pulley velocity : Outport  Port=3
  wires:
  Gain23/1 -> Minus2/3
  Gain4/1 -> Gain5/1
  [theta1] -> Gain24/1
  Gain11/1 -> Minus1/1
  [theta3_dot] -> Gain26/1
  Gain26/1 -> Minus2/5
  Gain22/1 -> Gain23/1
  Gain19/1 -> Minus2/1
  Gain21/1 -> Minus2/2
  Integrator/1 -> Integrator1/1, [theta1_dot], Gain8/1  "theta1_dot"
  Integrator1/1 -> Gain6/1, Gain2/1, [theta1]  "theta1"
  Integrator6/1 -> Integrator7/1, [x2_dot]  "x2_dot"
  Gain3/1 -> Minus/3
  Gain18/1 -> Gain19/1
  Gain1/1 -> Minus/4
  Gain2/1 -> Gain3/1
  Integrator2/1 -> [theta3_dot], Integrator4/1  "theta3_dot"
  Integrator4/1 -> Gain4/1, [theta3]  "theta3"
  [x2] -> Gain12/1
  Gain/1 -> Gain1/1
  Gain10/1 -> Gain11/1
  [theta1_dot] -> Divide1/3
  Gain24/1 -> Gain25/1
  Gain13/1 -> Minus1/3
  [theta3] -> Gain20/1
  [theta3] -> Gain14/1
  Gain15/1 -> Minus1/4
  Gain6/1 -> Gain7/1
  [theta3] -> Gain22/1
  Gain5/1 -> Minus/5
  [theta1] -> Gain10/1
  [x2] -> Gain18/1
  Minus2/1 -> Gain27/1
  Minus1/1 -> Gain17/1
  Minus/1 -> Gain9/1
  Gain7/1 -> Minus/2
  Integrator7/1 -> Gain/1, [x2]  "x2"
  Gain16/1 -> Minus1/5
  Gain8/1 -> Minus/1
  Gain17/1 -> Integrator6/1  "x2_dot_dot"
  Gain14/1 -> Gain15/1
  Gain20/1 -> Gain21/1
  Gain9/1 -> Integrator/1  "theta1_dot_dot"
  Gain12/1 -> Minus1/2
  Gain25/1 -> Minus2/4
  [x2] -> Gain13/1
  Minus3/1 -> Manual Switch/1  "Tourque"
  [x2_dot] -> Gain16/1
  [theta1_dot] -> drive pulley velocity/1
  [x2_dot] -> load velocity/1
  [theta3_dot] -> driven pulley velocity/1
  Gain27/1 -> Integrator2/1  "theta3_dot_dot"
  Voltage/1 -> Divide/1
  Constant/1 -> Divide/2, Divide1/1
  Constant2/1 -> Divide1/4, Divide/3
  Divide/1 -> Minus3/1
  Constant1/1 -> Divide1/2
  Divide1/1 -> Minus3/2
  Manual Switch/1 -> Minus/6
  DC Motor1/1(Tourque) -> Manual Switch/2  "Tourque"
  Pulse Generator11/1 -> DC Motor1/1(Voltage)
  [x2_dot] -> DC Motor1/2(Velocity)

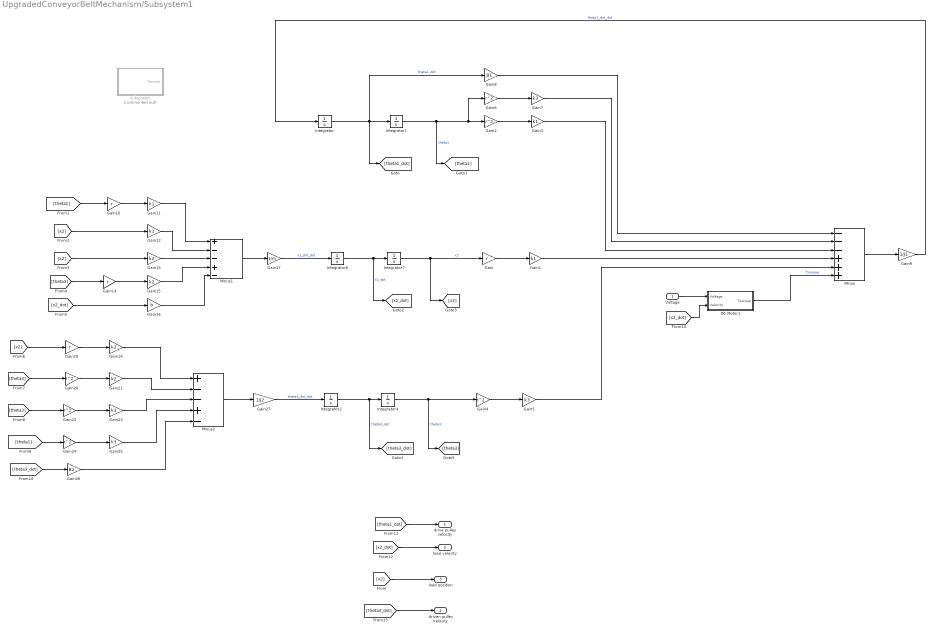
== system UpgradedConveyorBeltMechanism/Subsystem1 ==
  Voltage : Inport
  DC Motor1 : Subsystem
  Gain{,10,14,18} (4 alike) : Gain  Gain=r
  Gain{1,3,11..12} (4 alike) : Gain  Gain=k1
  Gain{13,15,19,21} (4 alike) : Gain  Gain=k2
  Gain16 : Gain  Gain=b
  Gain17 : Gain  Gain=1/m
  Gain{2,4,6,20,22,24} (6 alike) : Gain  Gain=r^2
  Gain{5,7,23,25} (4 alike) : Gain  Gain=k3
  Gain26 : Gain  Gain=B2
  Gain27 : Gain  Gain=1/J2
  Gain8 : Gain  Gain=B1
  Gain9 : Gain  Gain=1/J1
  Integrator{,1..2,4,6..7} (6 alike) : Integrator
  Minus : Sum  Inputs=---+++
  Minus1 : Sum  Inputs=+--+-
  Minus2 : Sum  Inputs=+--+-
  Subsystem : Subsystem  Commented=on
  drive pulley velocity : Outport
  load velocity : Outport  Port=2
  load position : Outport  Port=3
  driven pulley Velocity : Outport  Port=4
  wires:
  Gain23/1 -> Minus2/3
  Gain4/1 -> Gain5/1
  [theta1] -> Gain24/1
  Gain11/1 -> Minus1/1
  [theta3_dot] -> Gain26/1
  Gain26/1 -> Minus2/5
  Gain22/1 -> Gain23/1
  Gain19/1 -> Minus2/1
  Gain21/1 -> Minus2/2
  Integrator/1 -> Integrator1/1, [theta1_dot], Gain8/1  "theta1_dot"
  Integrator1/1 -> Gain6/1, Gain2/1, [theta1]  "theta1"
  Integrator6/1 -> Integrator7/1, [x2_dot]  "x2_dot"
  Gain3/1 -> Minus/3
  Gain18/1 -> Gain19/1
  Gain1/1 -> Minus/4
  Gain2/1 -> Gain3/1
  Integrator2/1 -> [theta3_dot], Integrator4/1  "theta3_dot"
  Integrator4/1 -> Gain4/1, [theta3]  "theta3"
  [x2] -> Gain12/1
  Gain/1 -> Gain1/1
  Gain10/1 -> Gain11/1
  Gain24/1 -> Gain25/1
  Gain13/1 -> Minus1/3
  [theta3] -> Gain20/1
  [theta3] -> Gain14/1
  Gain15/1 -> Minus1/4
  Gain6/1 -> Gain7/1
  [theta3] -> Gain22/1
  Gain5/1 -> Minus/5
  [theta1] -> Gain10/1
  [x2] -> Gain18/1
  Minus2/1 -> Gain27/1
  Minus1/1 -> Gain17/1
  Minus/1 -> Gain9/1
  Gain7/1 -> Minus/2
  Integrator7/1 -> Gain/1, [x2]  "x2"
  Gain16/1 -> Minus1/5
  Gain8/1 -> Minus/1
  Gain17/1 -> Integrator6/1  "x2_dot_dot"
  Gain14/1 -> Gain15/1
  Gain20/1 -> Gain21/1
  Gain9/1 -> Integrator/1  "theta1_dot_dot"
  Gain12/1 -> Minus1/2
  Gain25/1 -> Minus2/4
  [x2] -> Gain13/1
  [x2_dot] -> Gain16/1
  [theta1_dot] -> drive pulley velocity/1
  [x2_dot] -> load velocity/1
  Gain27/1 -> Integrator2/1  "theta3_dot_dot"
  DC Motor1/1(Tourque) -> Minus/6  "Tourque"
  [x2_dot] -> DC Motor1/2(Velocity)
  Voltage/1 -> DC Motor1/1(Voltage)
  [x2] -> load position/1
  [theta3_dot] -> driven pulley Velocity/1

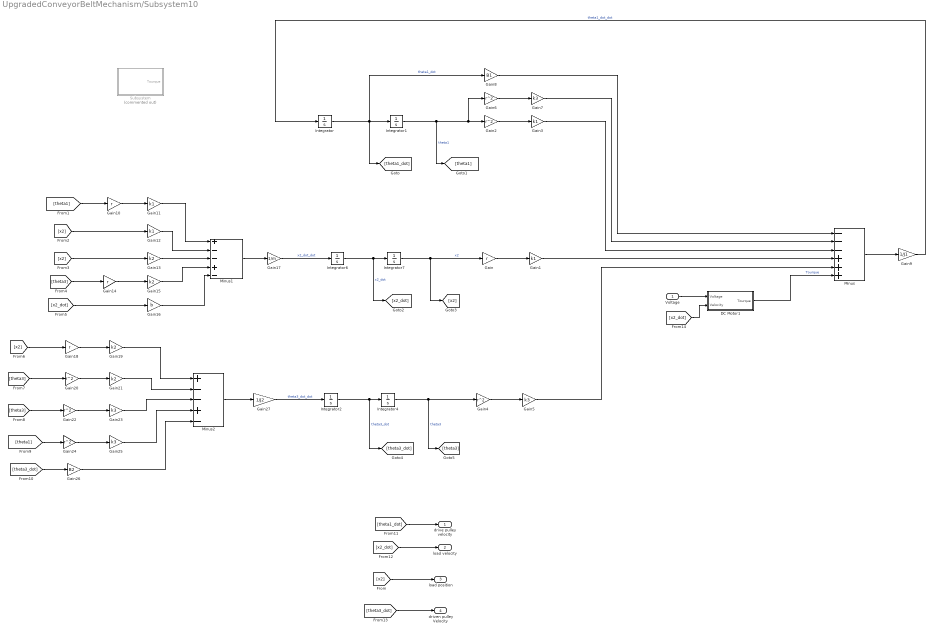
== system UpgradedConveyorBeltMechanism/Subsystem10 ==
  Voltage : Inport
  DC Motor1 : Subsystem
  Gain{,10,14,18} (4 alike) : Gain  Gain=r
  Gain{1,3,11..12} (4 alike) : Gain  Gain=k1
  Gain{13,15,19,21} (4 alike) : Gain  Gain=k2
  Gain16 : Gain  Gain=b
  Gain17 : Gain  Gain=1/m
  Gain{2,4,6,20,22,24} (6 alike) : Gain  Gain=r^2
  Gain{5,7,23,25} (4 alike) : Gain  Gain=k3
  Gain26 : Gain  Gain=B2
  Gain27 : Gain  Gain=1/J2
  Gain8 : Gain  Gain=B1
  Gain9 : Gain  Gain=1/J1
  Integrator{,1..2,4,6..7} (6 alike) : Integrator
  Minus : Sum  Inputs=---+++
  Minus1 : Sum  Inputs=+--+-
  Minus2 : Sum  Inputs=+--+-
  Subsystem : Subsystem  Commented=on
  drive pulley velocity : Outport
  load velocity : Outport  Port=2
  load position : Outport  Port=3
  driven pulley Velocity : Outport  Port=4
  wires:
  Gain23/1 -> Minus2/3
  Gain4/1 -> Gain5/1
  [theta1] -> Gain24/1
  Gain11/1 -> Minus1/1
  [theta3_dot] -> Gain26/1
  Gain26/1 -> Minus2/5
  Gain22/1 -> Gain23/1
  Gain19/1 -> Minus2/1
  Gain21/1 -> Minus2/2
  Integrator/1 -> Integrator1/1, [theta1_dot], Gain8/1  "theta1_dot"
  Integrator1/1 -> Gain6/1, Gain2/1, [theta1]  "theta1"
  Integrator6/1 -> Integrator7/1, [x2_dot]  "x2_dot"
  Gain3/1 -> Minus/3
  Gain18/1 -> Gain19/1
  Gain1/1 -> Minus/4
  Gain2/1 -> Gain3/1
  Integrator2/1 -> [theta3_dot], Integrator4/1  "theta3_dot"
  Integrator4/1 -> Gain4/1, [theta3]  "theta3"
  [x2] -> Gain12/1
  Gain/1 -> Gain1/1
  Gain10/1 -> Gain11/1
  Gain24/1 -> Gain25/1
  Gain13/1 -> Minus1/3
  [theta3] -> Gain20/1
  [theta3] -> Gain14/1
  Gain15/1 -> Minus1/4
  Gain6/1 -> Gain7/1
  [theta3] -> Gain22/1
  Gain5/1 -> Minus/5
  [theta1] -> Gain10/1
  [x2] -> Gain18/1
  Minus2/1 -> Gain27/1
  Minus1/1 -> Gain17/1
  Minus/1 -> Gain9/1
  Gain7/1 -> Minus/2
  Integrator7/1 -> Gain/1, [x2]  "x2"
  Gain16/1 -> Minus1/5
  Gain8/1 -> Minus/1
  Gain17/1 -> Integrator6/1  "x2_dot_dot"
  Gain14/1 -> Gain15/1
  Gain20/1 -> Gain21/1
  Gain9/1 -> Integrator/1  "theta1_dot_dot"
  Gain12/1 -> Minus1/2
  Gain25/1 -> Minus2/4
  [x2] -> Gain13/1
  [x2_dot] -> Gain16/1
  [theta1_dot] -> drive pulley velocity/1
  [x2_dot] -> load velocity/1
  Gain27/1 -> Integrator2/1  "theta3_dot_dot"
  DC Motor1/1(Tourque) -> Minus/6  "Tourque"
  [x2_dot] -> DC Motor1/2(Velocity)
  Voltage/1 -> DC Motor1/1(Voltage)
  [x2] -> load position/1
  [theta3_dot] -> driven pulley Velocity/1

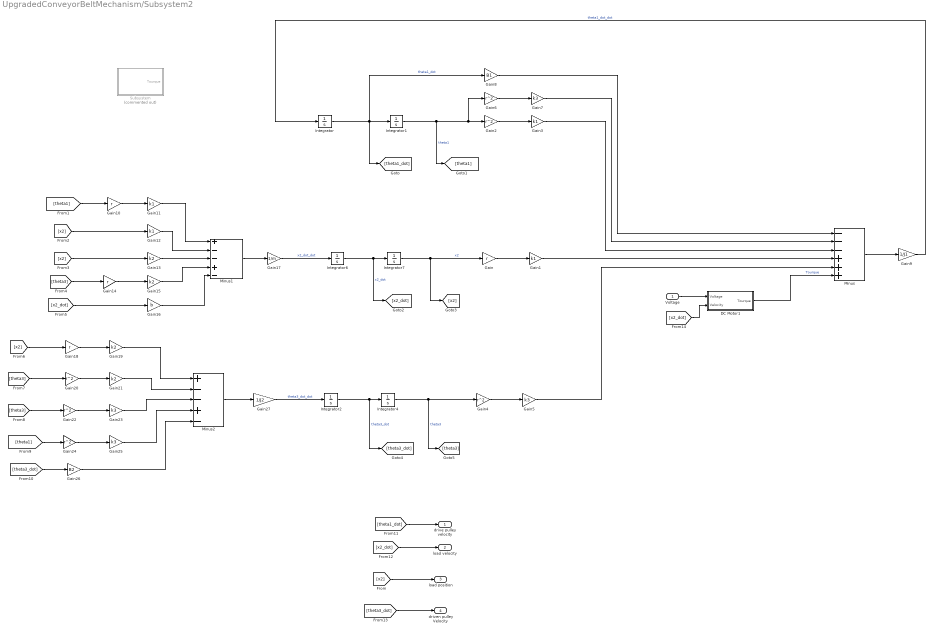
== system UpgradedConveyorBeltMechanism/Subsystem2 ==
  Voltage : Inport
  DC Motor1 : Subsystem
  Gain{,10,14,18} (4 alike) : Gain  Gain=r
  Gain{1,3,11..12} (4 alike) : Gain  Gain=k1
  Gain{13,15,19,21} (4 alike) : Gain  Gain=k2
  Gain16 : Gain  Gain=b
  Gain17 : Gain  Gain=1/m
  Gain{2,4,6,20,22,24} (6 alike) : Gain  Gain=r^2
  Gain{5,7,23,25} (4 alike) : Gain  Gain=k3
  Gain26 : Gain  Gain=B2
  Gain27 : Gain  Gain=1/J2
  Gain8 : Gain  Gain=B1
  Gain9 : Gain  Gain=1/J1
  Integrator{,1..2,4,6..7} (6 alike) : Integrator
  Minus : Sum  Inputs=---+++
  Minus1 : Sum  Inputs=+--+-
  Minus2 : Sum  Inputs=+--+-
  Subsystem : Subsystem  Commented=on
  drive pulley velocity : Outport
  load velocity : Outport  Port=2
  load position : Outport  Port=3
  driven pulley Velocity : Outport  Port=4
  wires:
  Gain23/1 -> Minus2/3
  Gain4/1 -> Gain5/1
  [theta1] -> Gain24/1
  Gain11/1 -> Minus1/1
  [theta3_dot] -> Gain26/1
  Gain26/1 -> Minus2/5
  Gain22/1 -> Gain23/1
  Gain19/1 -> Minus2/1
  Gain21/1 -> Minus2/2
  Integrator/1 -> Integrator1/1, [theta1_dot], Gain8/1  "theta1_dot"
  Integrator1/1 -> Gain6/1, Gain2/1, [theta1]  "theta1"
  Integrator6/1 -> Integrator7/1, [x2_dot]  "x2_dot"
  Gain3/1 -> Minus/3
  Gain18/1 -> Gain19/1
  Gain1/1 -> Minus/4
  Gain2/1 -> Gain3/1
  Integrator2/1 -> [theta3_dot], Integrator4/1  "theta3_dot"
  Integrator4/1 -> Gain4/1, [theta3]  "theta3"
  [x2] -> Gain12/1
  Gain/1 -> Gain1/1
  Gain10/1 -> Gain11/1
  Gain24/1 -> Gain25/1
  Gain13/1 -> Minus1/3
  [theta3] -> Gain20/1
  [theta3] -> Gain14/1
  Gain15/1 -> Minus1/4
  Gain6/1 -> Gain7/1
  [theta3] -> Gain22/1
  Gain5/1 -> Minus/5
  [theta1] -> Gain10/1
  [x2] -> Gain18/1
  Minus2/1 -> Gain27/1
  Minus1/1 -> Gain17/1
  Minus/1 -> Gain9/1
  Gain7/1 -> Minus/2
  Integrator7/1 -> Gain/1, [x2]  "x2"
  Gain16/1 -> Minus1/5
  Gain8/1 -> Minus/1
  Gain17/1 -> Integrator6/1  "x2_dot_dot"
  Gain14/1 -> Gain15/1
  Gain20/1 -> Gain21/1
  Gain9/1 -> Integrator/1  "theta1_dot_dot"
  Gain12/1 -> Minus1/2
  Gain25/1 -> Minus2/4
  [x2] -> Gain13/1
  [x2_dot] -> Gain16/1
  [theta1_dot] -> drive pulley velocity/1
  [x2_dot] -> load velocity/1
  Gain27/1 -> Integrator2/1  "theta3_dot_dot"
  DC Motor1/1(Tourque) -> Minus/6  "Tourque"
  [x2_dot] -> DC Motor1/2(Velocity)
  Voltage/1 -> DC Motor1/1(Voltage)
  [x2] -> load position/1
  [theta3_dot] -> driven pulley Velocity/1

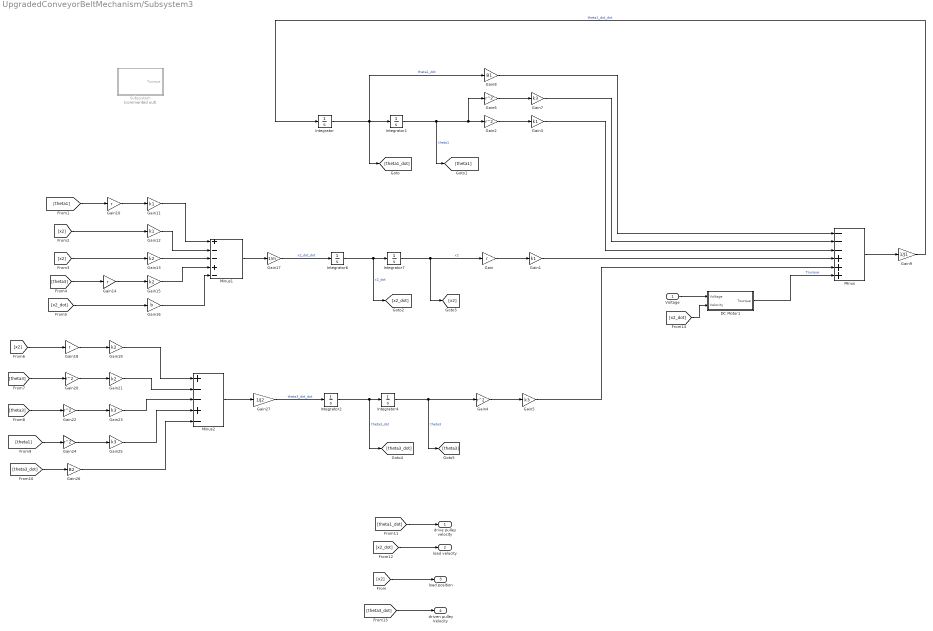
== system UpgradedConveyorBeltMechanism/Subsystem3 ==
  Voltage : Inport
  DC Motor1 : Subsystem
  Gain{,10,14,18} (4 alike) : Gain  Gain=r
  Gain{1,3,11..12} (4 alike) : Gain  Gain=k1
  Gain{13,15,19,21} (4 alike) : Gain  Gain=k2
  Gain16 : Gain  Gain=b
  Gain17 : Gain  Gain=1/m
  Gain{2,4,6,20,22,24} (6 alike) : Gain  Gain=r^2
  Gain{5,7,23,25} (4 alike) : Gain  Gain=k3
  Gain26 : Gain  Gain=B2
  Gain27 : Gain  Gain=1/J2
  Gain8 : Gain  Gain=B1
  Gain9 : Gain  Gain=1/J1
  Integrator{,1..2,4,6..7} (6 alike) : Integrator
  Minus : Sum  Inputs=---+++
  Minus1 : Sum  Inputs=+--+-
  Minus2 : Sum  Inputs=+--+-
  Subsystem : Subsystem  Commented=on
  drive pulley velocity : Outport
  load velocity : Outport  Port=2
  load position : Outport  Port=3
  driven pulley Velocity : Outport  Port=4
  wires:
  Gain23/1 -> Minus2/3
  Gain4/1 -> Gain5/1
  [theta1] -> Gain24/1
  Gain11/1 -> Minus1/1
  [theta3_dot] -> Gain26/1
  Gain26/1 -> Minus2/5
  Gain22/1 -> Gain23/1
  Gain19/1 -> Minus2/1
  Gain21/1 -> Minus2/2
  Integrator/1 -> Integrator1/1, [theta1_dot], Gain8/1  "theta1_dot"
  Integrator1/1 -> Gain6/1, Gain2/1, [theta1]  "theta1"
  Integrator6/1 -> Integrator7/1, [x2_dot]  "x2_dot"
  Gain3/1 -> Minus/3
  Gain18/1 -> Gain19/1
  Gain1/1 -> Minus/4
  Gain2/1 -> Gain3/1
  Integrator2/1 -> [theta3_dot], Integrator4/1  "theta3_dot"
  Integrator4/1 -> Gain4/1, [theta3]  "theta3"
  [x2] -> Gain12/1
  Gain/1 -> Gain1/1
  Gain10/1 -> Gain11/1
  Gain24/1 -> Gain25/1
  Gain13/1 -> Minus1/3
  [theta3] -> Gain20/1
  [theta3] -> Gain14/1
  Gain15/1 -> Minus1/4
  Gain6/1 -> Gain7/1
  [theta3] -> Gain22/1
  Gain5/1 -> Minus/5
  [theta1] -> Gain10/1
  [x2] -> Gain18/1
  Minus2/1 -> Gain27/1
  Minus1/1 -> Gain17/1
  Minus/1 -> Gain9/1
  Gain7/1 -> Minus/2
  Integrator7/1 -> Gain/1, [x2]  "x2"
  Gain16/1 -> Minus1/5
  Gain8/1 -> Minus/1
  Gain17/1 -> Integrator6/1  "x2_dot_dot"
  Gain14/1 -> Gain15/1
  Gain20/1 -> Gain21/1
  Gain9/1 -> Integrator/1  "theta1_dot_dot"
  Gain12/1 -> Minus1/2
  Gain25/1 -> Minus2/4
  [x2] -> Gain13/1
  [x2_dot] -> Gain16/1
  [theta1_dot] -> drive pulley velocity/1
  [x2_dot] -> load velocity/1
  Gain27/1 -> Integrator2/1  "theta3_dot_dot"
  DC Motor1/1(Tourque) -> Minus/6  "Tourque"
  [x2_dot] -> DC Motor1/2(Velocity)
  Voltage/1 -> DC Motor1/1(Voltage)
  [x2] -> load position/1
  [theta3_dot] -> driven pulley Velocity/1

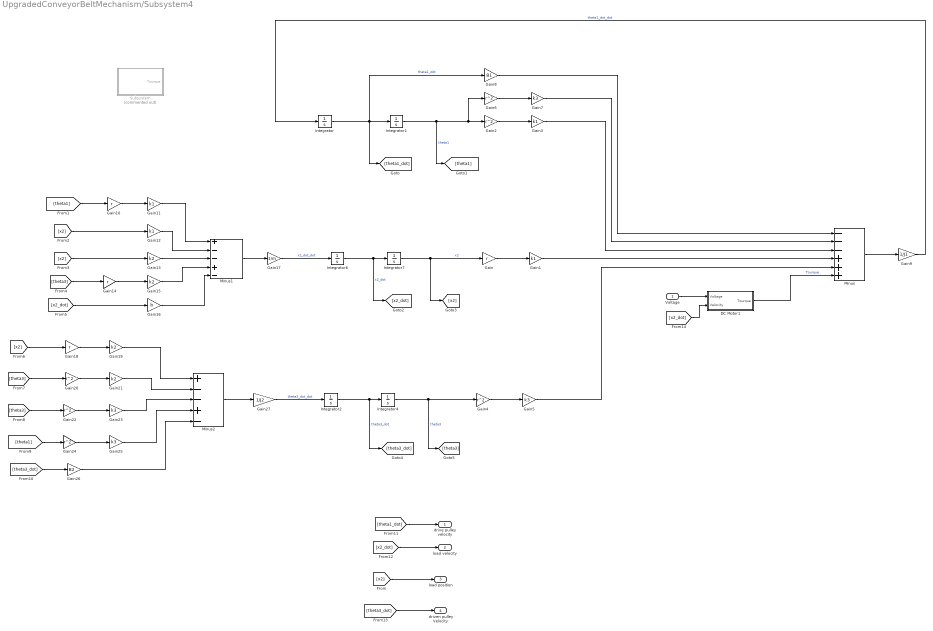
== system UpgradedConveyorBeltMechanism/Subsystem4 ==
  Voltage : Inport
  DC Motor1 : Subsystem
  Gain{,10,14,18} (4 alike) : Gain  Gain=r
  Gain{1,3,11..12} (4 alike) : Gain  Gain=k1
  Gain{13,15,19,21} (4 alike) : Gain  Gain=k2
  Gain16 : Gain  Gain=b
  Gain17 : Gain  Gain=1/m
  Gain{2,4,6,20,22,24} (6 alike) : Gain  Gain=r^2
  Gain{5,7,23,25} (4 alike) : Gain  Gain=k3
  Gain26 : Gain  Gain=B2
  Gain27 : Gain  Gain=1/J2
  Gain8 : Gain  Gain=B1
  Gain9 : Gain  Gain=1/J1
  Integrator{,1..2,4,6..7} (6 alike) : Integrator
  Minus : Sum  Inputs=---+++
  Minus1 : Sum  Inputs=+--+-
  Minus2 : Sum  Inputs=+--+-
  Subsystem : Subsystem  Commented=on
  drive pulley velocity : Outport
  load velocity : Outport  Port=2
  load position : Outport  Port=3
  driven pulley Velocity : Outport  Port=4
  wires:
  Gain23/1 -> Minus2/3
  Gain4/1 -> Gain5/1
  [theta1] -> Gain24/1
  Gain11/1 -> Minus1/1
  [theta3_dot] -> Gain26/1
  Gain26/1 -> Minus2/5
  Gain22/1 -> Gain23/1
  Gain19/1 -> Minus2/1
  Gain21/1 -> Minus2/2
  Integrator/1 -> Integrator1/1, [theta1_dot], Gain8/1  "theta1_dot"
  Integrator1/1 -> Gain6/1, Gain2/1, [theta1]  "theta1"
  Integrator6/1 -> Integrator7/1, [x2_dot]  "x2_dot"
  Gain3/1 -> Minus/3
  Gain18/1 -> Gain19/1
  Gain1/1 -> Minus/4
  Gain2/1 -> Gain3/1
  Integrator2/1 -> [theta3_dot], Integrator4/1  "theta3_dot"
  Integrator4/1 -> Gain4/1, [theta3]  "theta3"
  [x2] -> Gain12/1
  Gain/1 -> Gain1/1
  Gain10/1 -> Gain11/1
  Gain24/1 -> Gain25/1
  Gain13/1 -> Minus1/3
  [theta3] -> Gain20/1
  [theta3] -> Gain14/1
  Gain15/1 -> Minus1/4
  Gain6/1 -> Gain7/1
  [theta3] -> Gain22/1
  Gain5/1 -> Minus/5
  [theta1] -> Gain10/1
  [x2] -> Gain18/1
  Minus2/1 -> Gain27/1
  Minus1/1 -> Gain17/1
  Minus/1 -> Gain9/1
  Gain7/1 -> Minus/2
  Integrator7/1 -> Gain/1, [x2]  "x2"
  Gain16/1 -> Minus1/5
  Gain8/1 -> Minus/1
  Gain17/1 -> Integrator6/1  "x2_dot_dot"
  Gain14/1 -> Gain15/1
  Gain20/1 -> Gain21/1
  Gain9/1 -> Integrator/1  "theta1_dot_dot"
  Gain12/1 -> Minus1/2
  Gain25/1 -> Minus2/4
  [x2] -> Gain13/1
  [x2_dot] -> Gain16/1
  [theta1_dot] -> drive pulley velocity/1
  [x2_dot] -> load velocity/1
  Gain27/1 -> Integrator2/1  "theta3_dot_dot"
  DC Motor1/1(Tourque) -> Minus/6  "Tourque"
  [x2_dot] -> DC Motor1/2(Velocity)
  Voltage/1 -> DC Motor1/1(Voltage)
  [x2] -> load position/1
  [theta3_dot] -> driven pulley Velocity/1

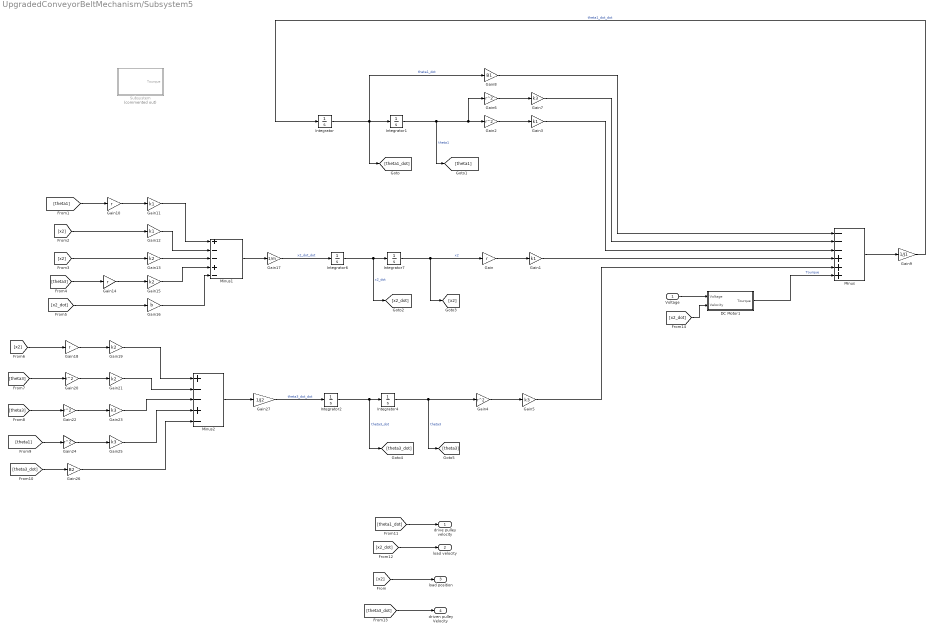
== system UpgradedConveyorBeltMechanism/Subsystem5 ==
  Voltage : Inport
  DC Motor1 : Subsystem
  Gain{,10,14,18} (4 alike) : Gain  Gain=r
  Gain{1,3,11..12} (4 alike) : Gain  Gain=k1
  Gain{13,15,19,21} (4 alike) : Gain  Gain=k2
  Gain16 : Gain  Gain=b
  Gain17 : Gain  Gain=1/m
  Gain{2,4,6,20,22,24} (6 alike) : Gain  Gain=r^2
  Gain{5,7,23,25} (4 alike) : Gain  Gain=k3
  Gain26 : Gain  Gain=B2
  Gain27 : Gain  Gain=1/J2
  Gain8 : Gain  Gain=B1
  Gain9 : Gain  Gain=1/J1
  Integrator{,1..2,4,6..7} (6 alike) : Integrator
  Minus : Sum  Inputs=---+++
  Minus1 : Sum  Inputs=+--+-
  Minus2 : Sum  Inputs=+--+-
  Subsystem : Subsystem  Commented=on
  drive pulley velocity : Outport
  load velocity : Outport  Port=2
  load position : Outport  Port=3
  driven pulley Velocity : Outport  Port=4
  wires:
  Gain23/1 -> Minus2/3
  Gain4/1 -> Gain5/1
  [theta1] -> Gain24/1
  Gain11/1 -> Minus1/1
  [theta3_dot] -> Gain26/1
  Gain26/1 -> Minus2/5
  Gain22/1 -> Gain23/1
  Gain19/1 -> Minus2/1
  Gain21/1 -> Minus2/2
  Integrator/1 -> Integrator1/1, [theta1_dot], Gain8/1  "theta1_dot"
  Integrator1/1 -> Gain6/1, Gain2/1, [theta1]  "theta1"
  Integrator6/1 -> Integrator7/1, [x2_dot]  "x2_dot"
  Gain3/1 -> Minus/3
  Gain18/1 -> Gain19/1
  Gain1/1 -> Minus/4
  Gain2/1 -> Gain3/1
  Integrator2/1 -> [theta3_dot], Integrator4/1  "theta3_dot"
  Integrator4/1 -> Gain4/1, [theta3]  "theta3"
  [x2] -> Gain12/1
  Gain/1 -> Gain1/1
  Gain10/1 -> Gain11/1
  Gain24/1 -> Gain25/1
  Gain13/1 -> Minus1/3
  [theta3] -> Gain20/1
  [theta3] -> Gain14/1
  Gain15/1 -> Minus1/4
  Gain6/1 -> Gain7/1
  [theta3] -> Gain22/1
  Gain5/1 -> Minus/5
  [theta1] -> Gain10/1
  [x2] -> Gain18/1
  Minus2/1 -> Gain27/1
  Minus1/1 -> Gain17/1
  Minus/1 -> Gain9/1
  Gain7/1 -> Minus/2
  Integrator7/1 -> Gain/1, [x2]  "x2"
  Gain16/1 -> Minus1/5
  Gain8/1 -> Minus/1
  Gain17/1 -> Integrator6/1  "x2_dot_dot"
  Gain14/1 -> Gain15/1
  Gain20/1 -> Gain21/1
  Gain9/1 -> Integrator/1  "theta1_dot_dot"
  Gain12/1 -> Minus1/2
  Gain25/1 -> Minus2/4
  [x2] -> Gain13/1
  [x2_dot] -> Gain16/1
  [theta1_dot] -> drive pulley velocity/1
  [x2_dot] -> load velocity/1
  Gain27/1 -> Integrator2/1  "theta3_dot_dot"
  DC Motor1/1(Tourque) -> Minus/6  "Tourque"
  [x2_dot] -> DC Motor1/2(Velocity)
  Voltage/1 -> DC Motor1/1(Voltage)
  [x2] -> load position/1
  [theta3_dot] -> driven pulley Velocity/1

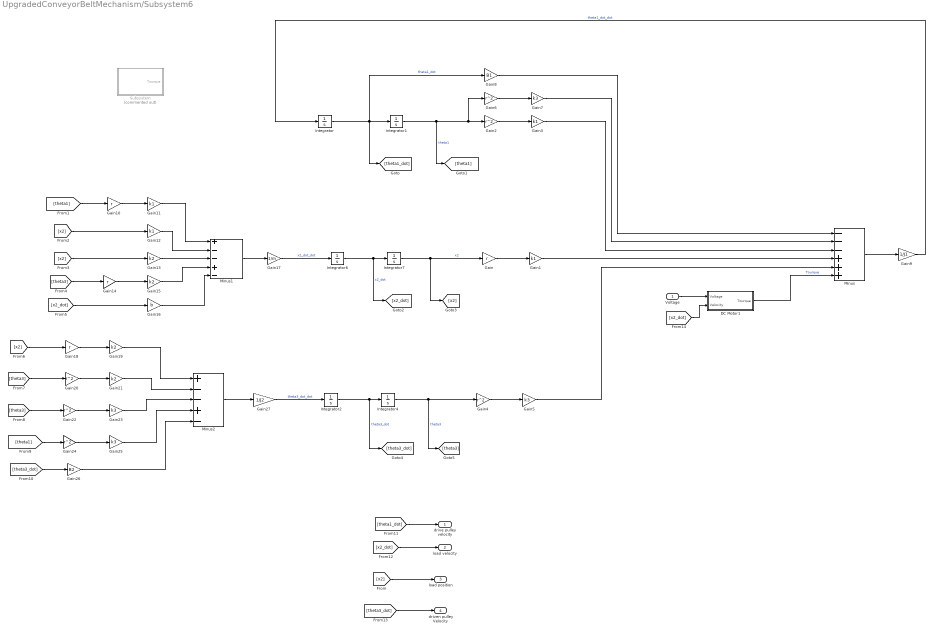
== system UpgradedConveyorBeltMechanism/Subsystem6 ==
  Voltage : Inport
  DC Motor1 : Subsystem
  Gain{,10,14,18} (4 alike) : Gain  Gain=r
  Gain{1,3,11..12} (4 alike) : Gain  Gain=k1
  Gain{13,15,19,21} (4 alike) : Gain  Gain=k2
  Gain16 : Gain  Gain=b
  Gain17 : Gain  Gain=1/m
  Gain{2,4,6,20,22,24} (6 alike) : Gain  Gain=r^2
  Gain{5,7,23,25} (4 alike) : Gain  Gain=k3
  Gain26 : Gain  Gain=B2
  Gain27 : Gain  Gain=1/J2
  Gain8 : Gain  Gain=B1
  Gain9 : Gain  Gain=1/J1
  Integrator{,1..2,4,6..7} (6 alike) : Integrator
  Minus : Sum  Inputs=---+++
  Minus1 : Sum  Inputs=+--+-
  Minus2 : Sum  Inputs=+--+-
  Subsystem : Subsystem  Commented=on
  drive pulley velocity : Outport
  load velocity : Outport  Port=2
  load position : Outport  Port=3
  driven pulley Velocity : Outport  Port=4
  wires:
  Gain23/1 -> Minus2/3
  Gain4/1 -> Gain5/1
  [theta1] -> Gain24/1
  Gain11/1 -> Minus1/1
  [theta3_dot] -> Gain26/1
  Gain26/1 -> Minus2/5
  Gain22/1 -> Gain23/1
  Gain19/1 -> Minus2/1
  Gain21/1 -> Minus2/2
  Integrator/1 -> Integrator1/1, [theta1_dot], Gain8/1  "theta1_dot"
  Integrator1/1 -> Gain6/1, Gain2/1, [theta1]  "theta1"
  Integrator6/1 -> Integrator7/1, [x2_dot]  "x2_dot"
  Gain3/1 -> Minus/3
  Gain18/1 -> Gain19/1
  Gain1/1 -> Minus/4
  Gain2/1 -> Gain3/1
  Integrator2/1 -> [theta3_dot], Integrator4/1  "theta3_dot"
  Integrator4/1 -> Gain4/1, [theta3]  "theta3"
  [x2] -> Gain12/1
  Gain/1 -> Gain1/1
  Gain10/1 -> Gain11/1
  Gain24/1 -> Gain25/1
  Gain13/1 -> Minus1/3
  [theta3] -> Gain20/1
  [theta3] -> Gain14/1
  Gain15/1 -> Minus1/4
  Gain6/1 -> Gain7/1
  [theta3] -> Gain22/1
  Gain5/1 -> Minus/5
  [theta1] -> Gain10/1
  [x2] -> Gain18/1
  Minus2/1 -> Gain27/1
  Minus1/1 -> Gain17/1
  Minus/1 -> Gain9/1
  Gain7/1 -> Minus/2
  Integrator7/1 -> Gain/1, [x2]  "x2"
  Gain16/1 -> Minus1/5
  Gain8/1 -> Minus/1
  Gain17/1 -> Integrator6/1  "x2_dot_dot"
  Gain14/1 -> Gain15/1
  Gain20/1 -> Gain21/1
  Gain9/1 -> Integrator/1  "theta1_dot_dot"
  Gain12/1 -> Minus1/2
  Gain25/1 -> Minus2/4
  [x2] -> Gain13/1
  [x2_dot] -> Gain16/1
  [theta1_dot] -> drive pulley velocity/1
  [x2_dot] -> load velocity/1
  Gain27/1 -> Integrator2/1  "theta3_dot_dot"
  DC Motor1/1(Tourque) -> Minus/6  "Tourque"
  [x2_dot] -> DC Motor1/2(Velocity)
  Voltage/1 -> DC Motor1/1(Voltage)
  [x2] -> load position/1
  [theta3_dot] -> driven pulley Velocity/1

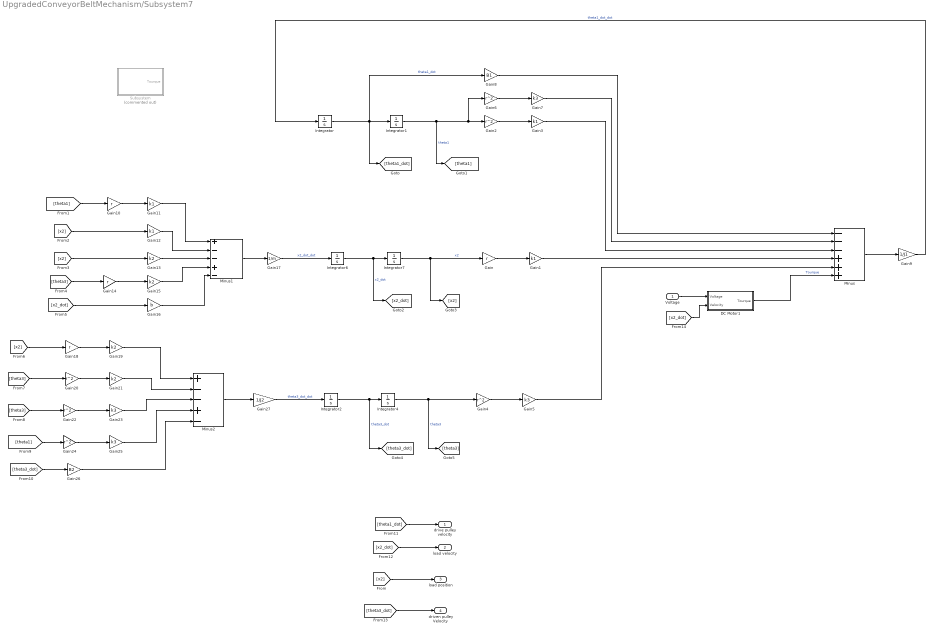
== system UpgradedConveyorBeltMechanism/Subsystem7 ==
  Voltage : Inport
  DC Motor1 : Subsystem
  Gain{,10,14,18} (4 alike) : Gain  Gain=r
  Gain{1,3,11..12} (4 alike) : Gain  Gain=k1
  Gain{13,15,19,21} (4 alike) : Gain  Gain=k2
  Gain16 : Gain  Gain=b
  Gain17 : Gain  Gain=1/m
  Gain{2,4,6,20,22,24} (6 alike) : Gain  Gain=r^2
  Gain{5,7,23,25} (4 alike) : Gain  Gain=k3
  Gain26 : Gain  Gain=B2
  Gain27 : Gain  Gain=1/J2
  Gain8 : Gain  Gain=B1
  Gain9 : Gain  Gain=1/J1
  Integrator{,1..2,4,6..7} (6 alike) : Integrator
  Minus : Sum  Inputs=---+++
  Minus1 : Sum  Inputs=+--+-
  Minus2 : Sum  Inputs=+--+-
  Subsystem : Subsystem  Commented=on
  drive pulley velocity : Outport
  load velocity : Outport  Port=2
  load position : Outport  Port=3
  driven pulley Velocity : Outport  Port=4
  wires:
  Gain23/1 -> Minus2/3
  Gain4/1 -> Gain5/1
  [theta1] -> Gain24/1
  Gain11/1 -> Minus1/1
  [theta3_dot] -> Gain26/1
  Gain26/1 -> Minus2/5
  Gain22/1 -> Gain23/1
  Gain19/1 -> Minus2/1
  Gain21/1 -> Minus2/2
  Integrator/1 -> Integrator1/1, [theta1_dot], Gain8/1  "theta1_dot"
  Integrator1/1 -> Gain6/1, Gain2/1, [theta1]  "theta1"
  Integrator6/1 -> Integrator7/1, [x2_dot]  "x2_dot"
  Gain3/1 -> Minus/3
  Gain18/1 -> Gain19/1
  Gain1/1 -> Minus/4
  Gain2/1 -> Gain3/1
  Integrator2/1 -> [theta3_dot], Integrator4/1  "theta3_dot"
  Integrator4/1 -> Gain4/1, [theta3]  "theta3"
  [x2] -> Gain12/1
  Gain/1 -> Gain1/1
  Gain10/1 -> Gain11/1
  Gain24/1 -> Gain25/1
  Gain13/1 -> Minus1/3
  [theta3] -> Gain20/1
  [theta3] -> Gain14/1
  Gain15/1 -> Minus1/4
  Gain6/1 -> Gain7/1
  [theta3] -> Gain22/1
  Gain5/1 -> Minus/5
  [theta1] -> Gain10/1
  [x2] -> Gain18/1
  Minus2/1 -> Gain27/1
  Minus1/1 -> Gain17/1
  Minus/1 -> Gain9/1
  Gain7/1 -> Minus/2
  Integrator7/1 -> Gain/1, [x2]  "x2"
  Gain16/1 -> Minus1/5
  Gain8/1 -> Minus/1
  Gain17/1 -> Integrator6/1  "x2_dot_dot"
  Gain14/1 -> Gain15/1
  Gain20/1 -> Gain21/1
  Gain9/1 -> Integrator/1  "theta1_dot_dot"
  Gain12/1 -> Minus1/2
  Gain25/1 -> Minus2/4
  [x2] -> Gain13/1
  [x2_dot] -> Gain16/1
  [theta1_dot] -> drive pulley velocity/1
  [x2_dot] -> load velocity/1
  Gain27/1 -> Integrator2/1  "theta3_dot_dot"
  DC Motor1/1(Tourque) -> Minus/6  "Tourque"
  [x2_dot] -> DC Motor1/2(Velocity)
  Voltage/1 -> DC Motor1/1(Voltage)
  [x2] -> load position/1
  [theta3_dot] -> driven pulley Velocity/1
